simulink model "Sensing"  (R2025b)
settings: configuration reference "code" (kept outside this file)
undefined symbols (not defined in the file or in its folder): TsSensors
settings Model: DataDictionary=test.sldd  Creator=rpumpo  LastModifiedBy=rpumpo
settings ConfigSetRef: SourceName=code

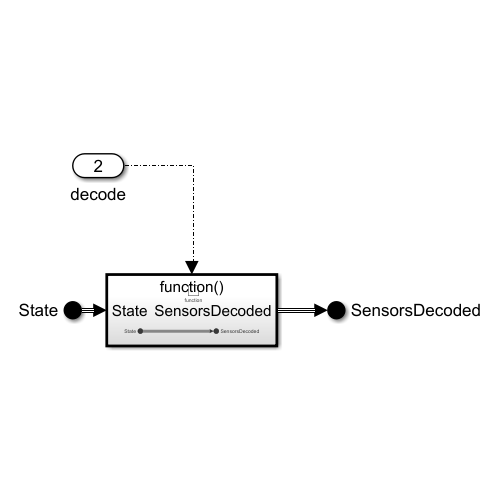
[thumbnail: Simulink's stored preview of the top-level diagram]
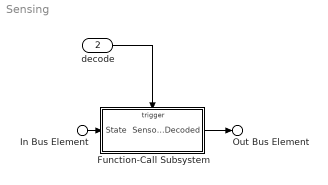
== system Sensing ==
  In Bus Element : Inport  PortName=State
  decode : Inport  Port=2  SampleTime=TsSensors  OutputFunctionCall=on
  Function-Call Subsystem : Subsystem  TreatAsAtomicUnit=on
  Out Bus Element : Outport  PortName=SensorsDecoded
  wires:
  In Bus Element/1 -> Function-Call Subsystem/1(State)
  Function-Call Subsystem/1(SensorsDecoded) -> Out Bus Element/1
  decode/1 -> Function-Call Subsystem/Trigger

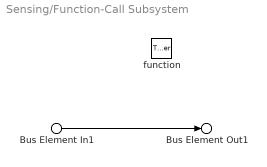
== system Sensing/Function-Call Subsystem ==
  Bus Element In1 : Inport  PortName=State
  function : TriggerPort  TriggerType=function-call  VariantControl=(inherit)
  Bus Element Out1 : Outport  PortName=SensorsDecoded
  wires:
  Bus Element In1/1 -> Bus Element Out1/1
